simulink model "hcu_main_ADASwEPS"  (Simulink 8.2)
settings: Solver=FixedStepDiscrete  StartTime=0.0  StopTime=inf  FixedStep=0.001  RelTol=1e-3
PostLoadFcn:
  | , if any(exist('dsrtsu_mdlpostloadfcn', 'file') == [2, 3, 6]), try dsrtsu_mdlpostloadfcn('Execute', bdroot); catch fprintf('Error in PostLoadFcn (dsrtsu_mdlpostloadfcn) for model "%s":\n %s\n', bdroot, lasterr); end, end,
values from neighbouring files (symbols this model uses):
  C_TASK_1MS_S = (	C_TICK_TIME_S       )    [hcu_local_hdr.m]    (also in temp_ovrd_values.m = double(	0.001                  ))
  C_TASK_5MS_S = (	C_TICK_TIME_S      	)    [hcu_local_hdr.m]
  ENUM_ADASLFCSTATUS_OFF = uint8(  0  )    [hcu_local_hdr.m]
  ENUM_ADASLFCSTATUS_STANDBY = uint8(  1  )    [hcu_local_hdr.m]
  ENUM_ADASLKASTATUS_ACTIVE = uint8(  2  )    [hcu_local_hdr.m]
  ENUM_ADASLKASTATUS_OFF = uint8(  0  )    [hcu_local_hdr.m]
  ENUM_ADASLKASTATUS_STANDBY = uint8(  1  )    [hcu_local_hdr.m]
  ENUM_EPSMODEREQ_ANGLE = uint8(  1  )    [hcu_local_hdr.m]
  ENUM_EPSMODEREQ_INTERNAL = uint8(  0  )    [hcu_local_hdr.m]
  ENUM_EPSMODEREQ_TORQUE = uint8(  2  )    [hcu_local_hdr.m]
  ENUM_GEARPOSN_1ST = uint8(  1  )    [hcu_local_hdr.m]
  ENUM_GEARPOSN_2ND = uint8(  2  )    [hcu_local_hdr.m]
  ENUM_GEARPOSN_3RD = uint8(  3  )    [hcu_local_hdr.m]
  ENUM_GEARPOSN_4TH = uint8(  4  )    [hcu_local_hdr.m]
  ENUM_GEARPOSN_5TH = uint8(  5  )    [hcu_local_hdr.m]
  ENUM_GEARPOSN_6TH = uint8(  6  )    [hcu_local_hdr.m]
  ENUM_GEARPOSN_PN = uint8(  0  )    [hcu_local_hdr.m]
  ENUM_GEARPOSN_R = uint8(  7  )    [hcu_local_hdr.m]
  FALSE = boolean( 0 )    [hcu_local_hdr.m]
  TRUE = boolean( 1 )    [hcu_local_hdr.m]
undefined symbols (not defined in the file or in its folder): AACC_DistCtrlIMult_X_mps2, AACC_DistCtrlPMult_X_mps2, AACC_GearActual_enum, AACC_SpdCtrlIMult_X_mps2, AACC_SpdCtrlPMult_X_mps2, AACC_VehSpd_kph, AISP_EPSCurrent_pct, AISP_TqASensorDelta_pct, AISP_TqBSensorDelta_pct, ENUM_ACCSTATUS_ACTIVE, ENUM_ACCSTATUS_OFF, ENUM_ACCSTATUS_STANDBY, ENUM_ADASLFCSTATUS_ACTIVE, ENUM_ADASLFCSTATUS_TRANSITION, ENUM_LFCCCONTSTATUS_ACTIVE, ENUM_LFCCCONTSTATUS_NOTAVAIL_TEMP, ENUM_LFCCCONTSTATUS_OFF, ENUM_LFCCCONTSTATUS_READY, ENUM_LFCCCONTSTATUS_TRANSITION, ENUM_LKACCONTSTATUS_ACTIVE, ENUM_LKACCONTSTATUS_NOTAVAIL_TEMP, ENUM_LKACCONTSTATUS_OFF, ENUM_LKACCONTSTATUS_READY, KACC_AcclReqMax_g, KACC_AcclReqMin_g, KACC_ACCSetTimeGapDef1_s, KACC_ACCSetTimeGapDef2_s, KACC_ACCSetTimeGapDef3_s, KACC_ACCSetTimeGapDef4_s, KACC_ACCSetTimeGapDef5_s, KACC_AirDensity_kgpm3, KACC_AirDragCoef_rat, KACC_CommandsOn_flg, KACC_CruzSpdChgTimeThres_s, KACC_DecReqSwOffThres_Nm, KACC_DecReqSwOnThres_Nm, KACC_DistCtrlAdjTime_s, KACC_DistCtrlCalRate_s, KACC_DistCtrlIC_mps2, KACC_DistCtrlIGain_rat, KACC_DistCtrlIMax_mps2, KACC_DistCtrlIMin_mps2, KACC_DistCtrlIRest_flg, KACC_DistCtrlKGain_rat, KACC_DistCtrlPause_flg, KACC_DistCtrlPGain_rat, KACC_FinalDriveEff_pct, KACC_FinalDriveRatio_rat, KACC_FrontalArea_m2, KACC_GearBoxEff_pct, KACC_LongPushSpdChg_kph, KACC_MaxAccSetSpd_kph, KACC_MinAccSetSpd_kph, KACC_SetAllowSpdLim_kph, KACC_SpdCtrlAdjTime_s, KACC_SpdCtrlCalRate_s, KACC_SpdCtrlIC_mps2, KACC_SpdCtrlIGain_rat, KACC_SpdCtrlIMax_mps2, KACC_SpdCtrlIMin_mps2 ... (+26)
libraries: simulink x54, adas_lib x6, rti1401lib_dio_type3 x4, rtimmsu_dsrtlib x3, hcu_lib x2, aeb x1, ddm x1, dfr x1, dgi x1, dhp x1, dinr x1, dip x1
(part 3 of 9)

== system hcu_main_ADASwEPS/Hw_In ==
  trig_Hw_In : TriggerPort  TriggerType=function-call
  ADC_TYPE4_BL1 : rti1401lib_adc_type4/ADC_TYPE4_BL1  DSProperties=struct('RTI',struct('Version',uint32(2),'BlockType',struct('isSLSource',uint8(1),'isSLSink',uint8(1),'isHWSource',uint8(0),'isHWSink',uint8(1),'isSetup',uint8(0),'isInline',uint8(1),'isNonInline',uint8(0),'isInterrupt',uint8(0),'isChannelwise',uint8(1)),'IOBoardType',{{'DS1401','STD','ADCT4'}},'UnitType','ADC','Identifier','ADC','DialogType','ML','BlockSet','NONE','SlaveProcessor','NONE'))  RTIBlockInterface=struct('InputPortsActive',0,'InputPortsWidth',int32(1),'InputPortsDataType',{{'SS_BOOLEAN'}},'InputPortsName',{{'Continue'}},'OutputPortsActive',[1 0],'OutputPortsWidth',int32([1 1]),'OutputPortsDataType',{{'SS_DOUBLE','SS_UINT8'}},'OutputPortsName',{{'ADC','Status'}},'DialogFcn','rti1401stdadct4adcgui','SampleTime',{{-1}},'InitLevel',3,'IconTransparency','on','BlockDisplay',{{['ADC TP4\nModule: 1\nChannel: 1'],'center'}},'BlockName',struct('Token',{{'ADC_TYPE4_BL1'}}))  RTIBlockParameters=struct('ADCSWStartDisable',{{0,'OFF',[0 1]}},'ModuleNo',{{1,'OFF',[1 16]}},'ChannelNo',{{1,'OFF',[1 16]}},'ConversionMode',{{1,'OFF',[1 2]}},'SampleMode',{{1,'OFF',[1 2]}},'TriggerSource',{{1,'OFF',[1 5]}},'EdgePolarity',{{1,'OFF',[1 2]}},'ConversionTriggerSource',{{2,'OFF',[1 6]}},'ConversionEdgePolarity',{{1,'OFF',[1 2]}},'ConversionPeriod',{{1e-06,'OFF',[]}},'ConversionPeriodCheck',{{0,'OFF',[]}},'BurstTriggerSource',{{1,'OFF',[1 6]}},'BurstEdgePolarity',{{1,'OFF',[1 2]}},'BurstSize',{{10,'OFF',[]}},'BurstSizeCheck',{{0,'OFF',[]}},'DataSetOffset',{{0,'OFF',[]}},'DataSetOffsetCheck',{{0,'OFF',[]}},'DataSetLength',{{1,'OFF',[]}},'DataSetLengthCheck',{{0,'OFF',[]}},'ReadMode',{{1,'OFF',[1 2]}},'SampleTime',{{-1,'OFF',[-1 inf]}},'SampleTimeCheck',{{1,'OFF',[]}},'StatusPortEnable',{{0,'OFF',[0 1]}},'VoltageRange',{{1,'OFF',[1 2]}},'TLCFileName',{{'rti1401adc_t4_adc','OFF',[]}})  RTISFcnParameters=struct('ADCSWStartDisable','int32','ModuleNo','int32','ChannelNo','int16','ConversionMode','int16','SampleMode','int16','TriggerSource','int16','EdgePolarity','int16','ConversionTriggerSource','int16','ConversionEdgePolarity','int16','ConversionPeriod','double','BurstTriggerSource','int16','BurstEdgePolarity','int16','BurstSize','int16','DataSetOffset','int16','DataSetLength','int16','ReadMode','int16','SampleTime','double','StatusPortEnable','int16','VoltageRange','int16','TLCFileName','char')  RTIBlockParaDefault=struct('ADCSWStartDisable',0,'ModuleNo',1,'ChannelNo',1,'ConversionMode',1,'SampleMode',1,'TriggerSource',1,'EdgePolarity',1,'ConversionTriggerSource',2,'ConversionEdgePolarity',1,'ConversionPeriod',1e-06,'ConversionPeriodCheck',0,'BurstTriggerSource',1,'BurstEdgePolarity',1,'BurstSize',10,'BurstSizeCheck',0,'DataSetOffset',0,'DataSetOffsetCheck',0,'DataSetLength',1,'DataSetLengthCheck',0,'ReadMode',1,'SampleTime',-1,'SampleTimeCheck',1,'StatusPortEnable',0,'VoltageRange',1,'TLCFileName','rti1401adc_t4_adc')
  Add : Sum
  DIO_TYPE3_ENC_BL1 : rti1401lib_dio_type3/DIO_TYPE3_ENC_BL1  DSProperties=struct('RTI',struct('Version',uint32(2),'BlockType',struct('isSLSource',uint8(1),'isSLSink',uint8(0),'isHWSource',uint8(1),'isHWSink',uint8(0),'isSetup',uint8(0),'isInline',uint8(1),'isNonInline',uint8(0),'isInterrupt',uint8(0),'isChannelwise',uint8(1)),'IOBoardType',{{'DS1401','STD','DIOT3'}},'UnitType','ENC','Identifier','ENC','DialogType','ML','BlockSet','NONE','SlaveProcessor','NONE'))  RTIBlockInterface=struct('OutputPortsWidth',int32([1 1]),'OutputPortsActive',[1 1],'OutputPortsName',{{'Position','Speed'}},'BlockDisplay',{{['DIO TP3 ENCODER\nModule: 1\nPort: 1\nChannel: 9'],'center'}},'IconTransparency','on','InitLevel',3,'DialogFcn','rti1401stddiot3encgui','BlockName',struct('Token',{{'DIO_TYPE3_ENC_BL1'}}))  RTIBlockParameters=struct('ModuleNo',{{1,'OFF',[1 16]}},'PortNo',{{1,'OFF',[1 3]}},'ChannelNo',{{9,'OFF',[1 15]}},'MinPosValue',{{'-2097152','ON',[-2097152 2097151.5]}},'MaxPosValue',{{'2097151.75','ON',[-2097151.75 2097151.75]}},'InitPosValue',{{'0','ON',[-2097152 2097151.75]}},'IndexSetMode',{{1,'OFF',[1 3]}},'IndexPosValue',{{'0','ON',[-2097152 2097151.75]}},'IndexGateMode',{{0,'OFF',[0 1]}},'NoiseFilter',{{1,'OFF',[1 8]}},'BuildCheckIndexMode',{{0,'OFF',[0 1]}},'TLCFileName',{{'rti1401dio_t3_enc','OFF',[]}},'EnableInterrupt',{{0,'OFF',[0 1]}},'TriggerEdgeType',{{1,'OFF',[1 3]}})  RTISFcnParameters=struct('ModuleNo','int32','PortNo','int16','ChannelNo','int16','MinPosValue','double','MaxPosValue','double','InitPosValue','double','IndexSetMode','int16','IndexPosValue','double','IndexGateMode','int16','NoiseFilter','int16','BuildCheckIndexMode','int16','TLCFileName','char','EnableInterrupt','int16','TriggerEdgeType','int32')  RTIBlockParaDefault=struct('ModuleNo',1,'PortNo',1,'ChannelNo',1,'MinPosValue',-2097152,'MaxPosValue',2097151.75,'InitPosValue',0,'IndexSetMode',1,'IndexPosValue',0,'IndexGateMode',0,'NoiseFilter',1,'BuildCheckIndexMode',0,'TLCFileName','rti1401dio_t3_enc','EnableInterrupt',0,'TriggerEdgeType',1)
  DIO_TYPE3_PWM2D_BL1 : rti1401lib_dio_type3/DIO_TYPE3_PWM2D_BL1  DSProperties=struct('RTI',struct('Version',uint32(2),'BlockType',struct('isSLSource',uint8(1),'isSLSink',uint8(0),'isHWSource',uint8(1),'isHWSink',uint8(0),'isSetup',uint8(0),'isInline',uint8(1),'isNonInline',uint8(0),'isInterrupt',uint8(0),'isChannelwise',uint8(1)),'IOBoardType',{{'DS1401','STD','DIOT3'}},'UnitType','PWM','Identifier','PWM2D','DialogType','ML','BlockSet','NONE','SlaveProcessor','NONE'))  RTIBlockInterface=struct('OutputPortsWidth',int32([1 1]),'OutputPortsActive',[1 1],'OutputPortsName',{{'Frequency',['Duty Cycle']}},'BlockDisplay',{{['DIO TP3 PWM2D\nModule: 1\nPort: 1\nChannel: 1'],'center'}},'IconTransparency','on','InitLevel',3,'DialogFcn','rti1401stddiot3pwm2dgui','BlockName',struct('Token',{{'DIO_TYPE3_PWM2D_BL1'}}))  RTIBlockParameters=struct('ModuleNo',{{1,'ON',[1 16]}},'PortNo',{{1,'OFF',[1 3]}},'ChannelNo',{{1,'ON',[1 16]}},'UpdateMode',{{2,'ON',[1 2]}},'FrequencyRange',{{1,'OFF',[1 16]}},'TLCFileName',{{'rti1401dio_t3_pwm2d','OFF',[]}},'EnableInterrupt',{{0,'OFF',[0 1]}},'TriggerEdgeType',{{3,'OFF',[1 3]}})  RTISFcnParameters=struct('ModuleNo','int32','PortNo','int16','ChannelNo','int16','UpdateMode','int16','FrequencyRange','int16','TLCFileName','char','EnableInterrupt','int16','TriggerEdgeType','int32')  RTIBlockParaDefault=struct('ModuleNo',1,'PortNo',1,'ChannelNo',1,'UpdateMode',1,'FrequencyRange',7,'TLCFileName','rti1401dio_t3_pwm2d','EnableInterrupt',0,'TriggerEdgeType',1)
  DIO_TYPE3_PWM2D_BL2 : rti1401lib_dio_type3/DIO_TYPE3_PWM2D_BL1  DSProperties=struct('RTI',struct('Version',uint32(2),'BlockType',struct('isSLSource',uint8(1),'isSLSink',uint8(0),'isHWSource',uint8(1),'isHWSink',uint8(0),'isSetup',uint8(0),'isInline',uint8(1),'isNonInline',uint8(0),'isInterrupt',uint8(0),'isChannelwise',uint8(1)),'IOBoardType',{{'DS1401','STD','DIOT3'}},'UnitType','PWM','Identifier','PWM2D','DialogType','ML','BlockSet','NONE','SlaveProcessor','NONE'))  RTIBlockInterface=struct('OutputPortsWidth',int32([1 1]),'OutputPortsActive',[1 1],'OutputPortsName',{{'Frequency',['Duty Cycle']}},'BlockDisplay',{{['DIO TP3 PWM2D\nModule: 1\nPort: 1\nChannel: 2'],'center'}},'IconTransparency','on','InitLevel',3,'DialogFcn','rti1401stddiot3pwm2dgui','BlockName',struct('Token',{{'DIO_TYPE3_PWM2D_BL1'}}))  RTIBlockParameters=struct('ModuleNo',{{1,'ON',[1 16]}},'PortNo',{{1,'OFF',[1 3]}},'ChannelNo',{{2,'ON',[1 16]}},'UpdateMode',{{2,'ON',[1 2]}},'FrequencyRange',{{1,'OFF',[1 16]}},'TLCFileName',{{'rti1401dio_t3_pwm2d','OFF',[]}},'EnableInterrupt',{{0,'OFF',[0 1]}},'TriggerEdgeType',{{1,'OFF',[1 3]}})  RTISFcnParameters=struct('ModuleNo','int32','PortNo','int16','ChannelNo','int16','UpdateMode','int16','FrequencyRange','int16','TLCFileName','char','EnableInterrupt','int16','TriggerEdgeType','int32')  RTIBlockParaDefault=struct('ModuleNo',1,'PortNo',1,'ChannelNo',1,'UpdateMode',1,'FrequencyRange',7,'TLCFileName','rti1401dio_t3_pwm2d','EnableInterrupt',0,'TriggerEdgeType',1)
  Delay : Delay  DelayLength=1  InitialCondition=1
  Delay1 : Delay  DelayLength=1  InitialCondition=1
  Divide : Product  Inputs=*/
  Divide1 : Product  Inputs=*/
  Divide3 : Product  Inputs=*/
  EPSEncCount_cnt : Constant  Value=36
  EPSGearRatio_rat : Constant  Value=20.5
  Gain1 : Gain  Gain=100
  Gain2 : Gain  Gain=100
  Gain3 : Gain  Gain=100
  Input_Bus : BusCreator  Inputs=6
  Interval Test : simulink/Logic and Bit Operations/Interval Test  IntervalClosedRight=on  uplimit=115  IntervalClosedLeft=on  lowlimit=95  OutDataTypeStr=boolean
  REV2DEG : Gain  Gain=360
  SEC2MIN : Gain  Gain=60
  Switch : Switch  Criteria=u2 ~= 0
  Switch1 : Switch  Criteria=u2 ~= 0
  Terminator3 : Terminator
  Terminator4 : Terminator
  Hw_In : Outport
  wires:
  ADC_TYPE4_BL1/1 -> Gain3/1
  Gain3/1 -> Input_Bus/1  "VHAL_EPSCurrent_pct"
  DIO_TYPE3_PWM2D_BL2/2 -> Gain2/1
  DIO_TYPE3_PWM2D_BL1/2 -> Gain1/1
  Gain1/1 -> Add/1, Switch/1
  DIO_TYPE3_PWM2D_BL1/1 -> Terminator3/1
  DIO_TYPE3_PWM2D_BL2/1 -> Terminator4/1
  Gain2/1 -> Add/2, Switch1/1
  SEC2MIN/1 -> Input_Bus/6  "VHAL_EPSMotorSpd_rpm"
  REV2DEG/1 -> Input_Bus/4, Divide3/1  "VHAL_EPSMotorAng_deg"
  Divide1/1 -> SEC2MIN/1
  Divide/1 -> REV2DEG/1
  EPSEncCount_cnt/1 -> Divide/2, Divide1/2
  DIO_TYPE3_ENC_BL1/2 -> Divide1/1
  DIO_TYPE3_ENC_BL1/1 -> Divide/1
  EPSGearRatio_rat/1 -> Divide3/2
  Divide3/1 -> Input_Bus/5  "VHAL_RelStrAng_deg"
  Input_Bus/1 -> Hw_In/1  "Hw_In"
  Add/1 -> Interval Test/1
  Switch/1 -> Delay/1, Input_Bus/2  "VHAL_TqSensorADuty_pct"
  Switch1/1 -> Delay1/1, Input_Bus/3  "VHAL_TqSensorBDuty_pct"
  Interval Test/1 -> Switch1/2, Switch/2
  Delay/1 -> Switch/3
  Delay1/1 -> Switch1/3

== system hcu_main_ADASwEPS/Hw_Out ==
  OSP_Out : Inport
  trig_Hw_Out : TriggerPort  TriggerType=function-call
  Bus Selector : BusSelector  OutputSignals=DAC_V,EPSDirection_flg
  DAC_TYPE3_M1_C1 : rti1401lib_dac_type3/DAC_TYPE3_M1_C1  ModuleNo=1  ChannelNo=1  VoltageInitValue=0  VoltageTermMode=off  VoltageTermValue=0  Reserved1=[]  Reserved2=[]  Reserved3=[]  Reserved4=[]  DSProperties=struct('RTI',struct('Version',uint32(1),'BlockType',struct('isSLSource',uint8(0),'isSLSink',uint8(1),'isHWSource',uint8(0),'isHWSink',uint8(1),'isSetup',uint8(0),'isInline',uint8(0),'isNonInline',uint8(1),'isInterrupt',uint8(0),'isChannelwise',uint8(1)),'IOBoardType',{{'DS1401','STD','DACT3'}},'UnitType','DAC','Identifier','DAC','DialogType','SL','BlockSet','NONE','SlaveProcessor','NONE'))  RTIBlockInterface=struct('InputPortsActive',1,'BlockDisplay',{{'DAC','center'}},'IconTransparency','off','InitLevel',1,'BlockName',struct('Token',{{'DAC_TYPE3_M','_C'}},'BlockParam',{{'ModuleNo','ChannelNo'}}),'MaskDescription',['Channel-wise write access to the 4 DAC channels'])  RTIBlockParameters=struct('ModuleNo',{{1,'ON',[1 16]}},'ChannelNo',{{1,'ON',[1 4]}},'VoltageInitValue',{{0,'ON',[0 4.5]}},'VoltageTermMode',{{logical(0),'ON',[0 1]}},'VoltageTermValue',{{0,'VoltageTermMode',[0 4.5]}})  RTISFcnParameters=struct('ModuleNo','double','ChannelNo','double','VoltageInitValue','double','VoltageTermMode','double','VoltageTermValue','double')  RTIBlockParaDefault=struct('ModuleNo',1,'ChannelNo',1,'VoltageInitValue',0,'VoltageTermMode',0,'VoltageTermValue',0)
  DIO_TYPE3_BIT_OUT_CH_BL1 : rti1401lib_dio_type3/DIO_TYPE3_BIT_OUT_CH_BL1  DSProperties=struct('RTI',struct('Version',uint32(2),'BlockType',struct('isSLSource',uint8(0),'isSLSink',uint8(1),'isHWSource',uint8(0),'isHWSink',uint8(1),'isSetup',uint8(0),'isInline',uint8(1),'isNonInline',uint8(0),'isInterrupt',uint8(0),'isChannelwise',uint8(1)),'IOBoardType',{{'DS1401','STD','DIOT3'}},'UnitType','BIT','Identifier','BITOUTCH','DialogType','ML','BlockSet','NONE','SlaveProcessor','NONE'))  RTIBlockInterface=struct('InputPortsWidth',int32(1),'InputPortsActive',1,'InputPortsDataType',{{'SS_BOOLEAN'}},'InputPortsName',{{'In'}},'BlockDisplay',{{['DIO TP3 BIT OUT\n Channelwise\nModule: 1\nPort: 1\nChannel: 1'],'center'}},'IconTransparency','on','InitLevel',3,'DialogFcn','rti1401stddiot3bitoutchgui','BlockName',struct('Token',{{'DIO_TYPE3_BIT_OUT_CH_BL1'}}))  RTIBlockParameters=struct('ModuleNo',{{1,'OFF',[1 16]}},'PortNo',{{1,'OFF',[1 3]}},'ChannelNo',{{1,'OFF',[1 16]}},'OutputStateInit',{{0,'OFF',[0 1]}},'TerminationMode',{{0,'OFF',[0 1]}},'OutputStateTermValidate',{{0,'OFF',[0 1]}},'OutputStateTerm',{{0,'OFF',[0 1]}},'SupplyRailsCh',{{[1 1],'OFF',[0 1 0 1]}},'TLCFileName',{{'rti1401dio_t3_bit_out_ch','OFF',[]}},'EnableInterrupt',{{0,'OFF',[0 1]}},'TriggerEdgeType',{{1,'OFF',[1 3]}})  RTISFcnParameters=struct('ModuleNo','int32','PortNo','int16','ChannelNo','int16','SupplyRailsCh','int16','OutputStateInit','int16','TerminationMode','int16','OutputStateTermValidate','int16','OutputStateTerm','int16','TLCFileName','char','EnableInterrupt','int16','TriggerEdgeType','int32')  RTIBlockParaDefault=struct('ModuleNo',1,'PortNo',1,'ChannelNo',1,'OutputStateInit',0,'TerminationMode',0,'OutputStateTermValidate',0,'OutputStateTerm',0,'SupplyRailsCh',[1 1],'TLCFileName','rti1401dio_t3_bit_out_ch','EnableInterrupt',0,'TriggerEdgeType',1)
  Data Type Conversion10 : DataTypeConversion
  Data Type Conversion2 : DataTypeConversion
  wires:
  Data Type Conversion10/1 -> DIO_TYPE3_BIT_OUT_CH_BL1/1
  Data Type Conversion2/1 -> DAC_TYPE3_M1_C1/1
  OSP_Out/1 -> Bus Selector/1
  Bus Selector/1 -> Data Type Conversion2/1  "<DAC_V>"
  Bus Selector/2 -> Data Type Conversion10/1  "<EPSDirection_flg>"

== system hcu_main_ADASwEPS/ISP ==
  Hw_In : Inport
  CAN_In : Inport  Port=2
  trig_ISP : TriggerPort  TriggerType=function-call
  AngleProcessing : Subsystem
  Bus Selector1 : BusSelector  OutputSignals=ABS2.VehSpeed,ADAS1.ADAS_StrAngReq_A,ADAS1.ADAS_StrAngReq,ADAS1.ADAS_LFCTransGain_A,ADAS1.ADAS_LFCTransGain,ABS4.LatAccel,ADAS1.ADAS_StrTqReq_A,ADAS1.ADAS_StrTqReq,ADAS1.ADAS_EPSMode,ADAS1.ADAS_LKAStatus,ADAS1.ADAS_LFCMode,ADAS1.ADAS_LFCStatus
  Bus Selector2 : BusSelector  OutputSignals=VHAL_EPSCurrent_pct
  Bus Selector3 : BusSelector  OutputSignals=VHAL_TqSensorADuty_pct,VHAL_TqSensorBDuty_pct
  Bus Selector4 : BusSelector  OutputSignals=VHAL_RelStrAng_deg
  Bus Selector5 : BusSelector  OutputSignals=VHAL_RelStrAng_deg
  Bus Selector6 : BusSelector  OutputSignals=ABS2.VehSpeed,ABS4.YawRate,ABS4.YawRate_V,ABS3.LR_RawWhlSpeed,ABS3.LR_RawWhlSpeed_V,ABS3.RR_RawWhlSpeed,ABS3.RR_RawWhlSpeed_V
  Bus Selector7 : BusSelector  OutputSignals=VHAL_EPSMotorSpd_rpm,VHAL_RelStrAng_deg
  ISP_Bus : BusCreator  Inputs=21
  KISP_EPSZeroReset_flg : Constant  Value=0
  Logical Operator1 : Logic  Operator=NOT  AllPortsSameDT=off  OutDataTypeStr=boolean
  Logical Operator2 : Logic  Operator=NOT  AllPortsSameDT=off  OutDataTypeStr=boolean
  Logical Operator3 : Logic  Operator=NOT  AllPortsSameDT=off  OutDataTypeStr=boolean
  MISP_EPSCurrent_A : Lookup  InputValues=AISP_EPSCurrent_pct  Table=MISP_EPSCurrent_A  LookUpMeth=Interpolation-Use End Values
      settings: AttributesFormatString="Input=\"%<InputValues>\"\\nOutput=\"%<Table>\""
  PassThrough : Subsystem
  TqProcessing : Subsystem
  ISP_Out : Outport
  wires:
  MISP_EPSCurrent_A/1 -> ISP_Bus/1  "VISP_EPSCurrent_A"
  KISP_EPSZeroReset_flg/1 -> AngleProcessing/1(KISP_EPSZeroReset_flg), TqProcessing/3(KISP_EPSZeroReset_flg)
  Hw_In/1 -> Bus Selector3/1, Bus Selector4/1, [Hw_In], Bus Selector2/1
  ISP_Bus/1 -> ISP_Out/1
  CAN_In/1 -> [CAN_In], Bus Selector1/1
  TqProcessing/1(VISP_EPSTqOnShaft_Nm) -> ISP_Bus/2
  TqProcessing/2(VISP_EPSTqOnShaftValid_flg) -> ISP_Bus/3
  AngleProcessing/1(VISP_StrAng_deg) -> ISP_Bus/4
  AngleProcessing/2(VISP_StrAngValid_flg) -> ISP_Bus/5
  Bus Selector1/1 -> PassThrough/2(VHAL_VehSpd_kph)  "<VehSpeed>"
  Logical Operator2/1 -> AngleProcessing/5(VHAL_YawRateValid_flg)
  Logical Operator3/1 -> AngleProcessing/9(VHAL_RRRawWhlSpdValid_flg)
  Logical Operator1/1 -> AngleProcessing/7(VHAL_LRRawWhlSpdValid_flg)
  PassThrough/1(VISP_StrAngSensorValid_flg) -> ISP_Bus/6
  Bus Selector1/3 -> PassThrough/4(VHAL_StrAngReq_deg)  "<ADAS_StrAngReq>"
  Bus Selector1/2 -> PassThrough/3(VHAL_StrAngReqAppl_flg)  "<ADAS_StrAngReq_A>"
  PassThrough/3(VISP_StrAngReq_deg) -> ISP_Bus/8
  PassThrough/2(VISP_StrAngReqAppl_flg) -> ISP_Bus/7
  PassThrough/4(VISP_VehSpd_kph) -> ISP_Bus/9
  PassThrough/5(VISP_RelStrAng_deg) -> ISP_Bus/10
  Bus Selector1/5 -> PassThrough/6(VHAL_LFCTransGain_rat)  "<ADAS_LFCTransGain>"
  Bus Selector1/4 -> PassThrough/5(VHAL_LFCTransGainAppl_flg)  "<ADAS_LFCTransGain_A>"
  PassThrough/7(VISP_LFCTransGain_rat) -> ISP_Bus/12
  PassThrough/6(VISP_LFCTransGainAppl_flg) -> ISP_Bus/11
  Bus Selector1/6 -> PassThrough/7(VHAL_LatAccel_mps2)  "<LatAccel>"
  PassThrough/8(VISP_LatAccel_mps2) -> ISP_Bus/13
  Bus Selector1/7 -> PassThrough/8(VHAL_StrTqReqAppl_flg)  "<ADAS_StrTqReq_A>"
  Bus Selector1/8 -> PassThrough/9(VHAL_StrTqReq_Nm)  "<ADAS_StrTqReq>"
  PassThrough/9(VISP_StrTqReqAppl_flg) -> ISP_Bus/14
  PassThrough/10(VISP_StrTqReq_Nm) -> ISP_Bus/15
  PassThrough/15(VISP_EPSMotorSpd_rpm) -> ISP_Bus/20
  PassThrough/16(VISP_EPSMotorAng_deg) -> ISP_Bus/21
  Bus Selector2/1 -> MISP_EPSCurrent_A/1  "<VHAL_EPSCurrent_pct>"
  Bus Selector3/1 -> TqProcessing/1(VHAL_TqSensorADuty_pct)  "<VHAL_TqSensorADuty_pct>"
  Bus Selector3/2 -> TqProcessing/2(VHAL_TqSensorBDuty_pct)  "<VHAL_TqSensorBDuty_pct>"
  Bus Selector4/1 -> AngleProcessing/2(VHAL_RelStrAng_deg)  "<VHAL_RelStrAng_deg>"
  Bus Selector5/1 -> PassThrough/1(VHAL_RelStrAng_deg)  "<VHAL_RelStrAng_deg>"
  [Hw_In] -> Bus Selector5/1
  [CAN_In] -> Bus Selector6/1
  Bus Selector6/1 -> AngleProcessing/3(VHAL_VehSpd_kph)  "<VehSpeed>"
  Bus Selector6/2 -> AngleProcessing/4(VHAL_YawRate_degps)  "<YawRate>"
  Bus Selector6/3 -> Logical Operator2/1  "<YawRate_V>"
  Bus Selector6/4 -> AngleProcessing/6(VHAL_LRRawWhlSpd_kph)  "<LR_RawWhlSpeed>"
  Bus Selector6/5 -> Logical Operator1/1  "<LR_RawWhlSpeed_V>"
  Bus Selector6/6 -> AngleProcessing/8(VHAL_RRRawWhlSpd_kph)  "<RR_RawWhlSpeed>"
  Bus Selector6/7 -> Logical Operator3/1  "<RR_RawWhlSpeed_V>"
  [Hw_In] -> Bus Selector7/1
  Bus Selector7/1 -> PassThrough/14(VHAL_EPSMotorSpd_rpm)  "<VHAL_EPSMotorSpd_rpm>"
  Bus Selector7/2 -> PassThrough/15(VHAL_EPSMotorAng_deg)  "<VHAL_RelStrAng_deg>"
  Bus Selector1/9 -> PassThrough/10(VHAL_EPSModeReq_enum)  "<ADAS_EPSMode>"
  Bus Selector1/10 -> PassThrough/11(VHAL_ADASLKAStatus_enum)  "<ADAS_LKAStatus>"
  Bus Selector1/11 -> PassThrough/12(VHAL_ADASLFCMode_enum)  "<ADAS_LFCMode>"
  Bus Selector1/12 -> PassThrough/13(VHAL_ADASLFCStatus_enum)  "<ADAS_LFCStatus>"
  PassThrough/11(VISP_EPSModeReq_enum) -> ISP_Bus/16
  PassThrough/12(VISP_ADASLKAStatus_enum) -> ISP_Bus/17
  PassThrough/13(VISP_ADASLFCMode_enum) -> ISP_Bus/18
  PassThrough/14(VISP_ADASLFCStatus_enum) -> ISP_Bus/19

== system hcu_main_ADASwEPS/OSP ==
  BISP_outputs : Inport
  BEPSS_outputs : Inport  Port=2
  trig_OSP : TriggerPort  TriggerType=function-call
  Abs : Abs
  Bus Creator : BusCreator  Inputs=2
  Bus Selector : BusSelector  OutputSignals=VOSP_MotorDuty_pct
  Compare To Zero : simulink/Logic and Bit Operations/Compare To Zero  relop=>=  OutDataTypeStr=boolean
  Gain3 : Gain  Gain=1/100*4.5
  Negative : Constant  OutDataTypeStr=boolean
  OSP : Subsystem
  Positive : Constant  Value=0  OutDataTypeStr=boolean
  Switch : Switch  Criteria=u2 ~= 0
  OSP_Out : Outport
  BOSP_outputs : Outport  Port=2
  wires:
  Gain3/1 -> Bus Creator/1  "DAC_V"
  Positive/1 -> Switch/1
  Negative/1 -> Switch/3
  Compare To Zero/1 -> Switch/2
  Switch/1 -> Bus Creator/2  "EPSDirection_flg"
  Abs/1 -> Gain3/1
  Bus Creator/1 -> OSP_Out/1  "OSP_Out"
  BEPSS_outputs/1 -> OSP/2(BEPSS_outputs)
  Bus Selector/1 -> Compare To Zero/1, Abs/1  "<VOSP_MotorDuty_pct>"
  OSP/1(BOSP_outputs) -> BOSP_outputs/1, Bus Selector/1
  BISP_outputs/1 -> OSP/1(BISP_outputs)

== system hcu_main_ADASwEPS/RTI Data ==
  RTI Data Store : Subsystem  Tag="struct('private',struct('version',struct('dsVer',uint32(2),'dsVerCreation',uint32(2),'RTI',struct('ver','7.4','type','RTI1401')),'access',struct('type','Model','isPerm',1,'created',['17-Nov-2015 11:37:15'],'modified',['31-Jan-2016 23:13:02'],'location','')),'public',struct('main',struct('data',[]),'sub',struct('name',{{'hcu_main_ADASwEPS'}},'data',{{struct('TH',struct('thTaskInfo',struct('taskType',{'TIMER','HWINT','TMRINT','SWINT','GLINT'},'tasksNumOf',{1,1,0,0,0},'srcIds',{{'TIMERA'},{'BB_BYP_ETHT1M0I0S0'},{},{},{}},'taskNames',{{['Timer Task 1']},{['rti_ethernet_interface_name Interrupt [RX/TX]']},{},{},{}})),'th_tc',struct('dataType',{'TASK','TASK'},'taskGroupId',{'',''},'taskGroupList',{{},{}},'taskSchedulingPolicy',{'FCFS','FCFS'},'taskType',{'TIMER','HWINT'},'blkh',{-1,['hcu_main_ADASwEPS/ETHERNET_UDP_SETUP_BL1/Common Hardware' char(10) 'Interrupt Interface']},'srcId',{'TIMERA','BB_BYP_ETHT1M0I0S0'},'srcSgnName',{['Timer A interrupt'],['BB_BYP_ETH Type 1 Module 1 HW-Int 0 Interrupt 0']},'srcCpuName',{'',''},'taskName',{['Timer Task 1  [0.001] s'],['rti_ethernet_interface_name Interrupt [RX/TX]']},'taskNameDisplayExt',{'',''},'smplTime',{0.001,0},'smplTimeOffs',{0,0},'hasFixedPriority',{0,0},'priority',{1,2},'hasFixedOvc',{0,0},'ovcType',{1,1},'ovcMax',{1,1}),'tc_th',struct('dataType',{'TASK','TASK'},'taskGroupId',{'',''},'taskGroupList',{{},{}},'taskSchedulingPolicy',{'FCFS','FCFS'},'taskType',{'TIMER','HWINT'},'blkh',{-1,['hcu_main_ADASwEPS/ETHERNET_UDP_SETUP_BL1/Common Hardware' char(10) 'Interrupt Interface']},'srcId',{'TIMERA','BB_BYP_ETHT1M0I0S0'},'srcSgnName',{['Timer A interrupt'],['BB_BYP_ETH Type 1 Module 1 HW-Int 0 Interrupt 0']},'srcCpuName',{'',''},'taskName',{['Timer Task 1  [0.001] s'],['rti_ethernet_interface_name Interrupt [RX/TX]']},'taskNameDisplayExt',{'',''},'smplTime',{0.001,0},'smplTimeOffs',{0,0},'hasFixedPriority',{0,0},'priority',{1,2},'hasFixedOvc',{0,0},'ovcType',{1,1},'ovcMax',{1,1}))}})))"  mask(RTI_DATA_STORE){}
      mask help:
      | RTI Data Store Block. This block is used by RTI to store internal model dependent data. Deleting this block will result in data loss.
      |
      | NEVER DELETE, COPY, OR MODIFY THIS BLOCK!
      mask Help:
      | RTI Data Store Block. This block is used by RTI to store internal model dependent data. Deleting this block will result in data loss.
      | 
      | NEVER DELETE, COPY, OR MODIFY THIS BLOCK!
      mask Display: text(0.5, 0.5, ' ', 'HorizontalAlignment', 'center');

== system hcu_main_ADASwEPS/RTICANMM ControllerSetup ==
  VariationInput : Inport
  Reset : Inport  Port=2
  ModelClose : Subsystem  mask(RTICANMMModelClose){}
  RTICANMMCHANNEL_TLC : S-Function  FunctionName=rticanmm_tlc_adv  Parameters=1401,1,1,0,500,14011143421  EnableBusSupport=off  mask(RTICANMMCHANNEL_TLC){}
  Variation_DTC : DataTypeConversion  SaturateOnIntegerOverflow=on  RndMeth=Zero
  sfcn : S-Function  InitFcn=rticanmm_initfcn(gcb, 'SFCNs')  FunctionName=RTICANMM_SETUP_CAN_1  EnableBusSupport=off
      mask init:
      | rticanmm_initfcn(gcb, 'SFCNs')
  wires:
  Reset/1 -> sfcn/2
  VariationInput/1 -> Variation_DTC/1
  Variation_DTC/1 -> sfcn/1

== system hcu_main_ADASwEPS/RTICANMM ControllerSetup1 ==
  VariationInput : Inport
  Reset : Inport  Port=2
  ModelClose : Subsystem  mask(RTICANMMModelClose){}
  RTICANMMCHANNEL_TLC : S-Function  FunctionName=rticanmm_tlc_adv  Parameters=1401,1,2,0,500,14011243421  EnableBusSupport=off  mask(RTICANMMCHANNEL_TLC){}
  Variation_DTC : DataTypeConversion  SaturateOnIntegerOverflow=on  RndMeth=Zero
  sfcn : S-Function  InitFcn=rticanmm_initfcn(gcb, 'SFCNs')  FunctionName=RTICANMM_SETUP_CAN_2  EnableBusSupport=off
      mask init:
      | rticanmm_initfcn(gcb, 'SFCNs')
  wires:
  Reset/1 -> sfcn/2
  VariationInput/1 -> Variation_DTC/1
  Variation_DTC/1 -> sfcn/1

== system hcu_main_ADASwEPS/RTICANMM GeneralSetup ==
  ModelClose : Subsystem  mask(RTICANMMModelClose){}
  TRC Exclusion : rtimmsu_dsrtlib/TRC Exclusion

== system hcu_main_ADASwEPS/User2CAN1__ ==
  BOSP_outputs : Inport
  BOUTP_outputs : Inport  Port=2  OutDataTypeStr=Bus: BOUTP_outputs
  ADAS1 : Subsystem
  ADAS2 : Subsystem
  ADAS3 : Subsystem
  ADAS4 : Subsystem
  ADAS5 : Subsystem
  EPAS2 : Subsystem
  EPAS3 : Subsystem
  SAS1 : Subsystem
  buscreator : BusCreator  Inputs=8
  out : Outport
  wires:
  ADAS1/1(out) -> buscreator/1  "ADAS1"
  ADAS2/1(out) -> buscreator/2  "ADAS2"
  ADAS3/1(out) -> buscreator/3  "ADAS3"
  ADAS4/1(out) -> buscreator/4  "ADAS4"
  ADAS5/1(out) -> buscreator/5  "ADAS5"
  EPAS2/1(out) -> buscreator/6  "EPAS2"
  EPAS3/1(out) -> buscreator/7  "EPAS3"
  SAS1/1(out) -> buscreator/8  "SAS1"
  buscreator/1 -> out/1  "CAN"
  BOUTP_outputs/1 -> ADAS1/1(BOUTP_outputs), ADAS2/1(BOUTP_outputs), ADAS3/1(BOUTP_outputs), ADAS5/1(BOUTP_outputs), ADAS4/1(BOUTP_outputs)
  BOSP_outputs/1 -> SAS1/1(BOSP_outputs), EPAS3/1(BOSP_outputs), EPAS2/1(BOSP_outputs)

== system hcu_main_ADASwEPS/User2RTICANMM MainBlock_ ==
  CAN1_Rx : Inport
  ABS2_C : Subsystem
  ABS4_C : Subsystem
  SAS1_C : Subsystem
  SpeedInformation : Subsystem
  YawRateInformation : Subsystem
  buscreator : BusCreator  Inputs=5
  out : Outport
  wires:
  ABS2_C/1(out) -> buscreator/1  "ABS2_C"
  ABS4_C/1(out) -> buscreator/2  "ABS4_C"
  SAS1_C/1(out) -> buscreator/3  "SAS1_C"
  SpeedInformation/1(out) -> buscreator/4  "SpeedInformation"
  YawRateInformation/1(out) -> buscreator/5  "YawRateInformation"
  buscreator/1 -> out/1  "CAN"
  CAN1_Rx/1 -> YawRateInformation/1(CAN1_Rx), SpeedInformation/1(CAN1_Rx), SAS1_C/1(CAN1_Rx), ABS4_C/1(CAN1_Rx), ABS2_C/1(CAN1_Rx1)

== system hcu_main_ADASwEPS/APPH/ACC ==
  BDINR_outputs : Inport  OutDataTypeStr=Bus: BDINR_outputs
  BMCT_outputs : Inport  Port=2  OutDataTypeStr=Bus: BMCT_outputs
  BAEB_outputs : Inport  Port=3  OutDataTypeStr=Bus: BAEB_outputs
  trig_ACC : TriggerPort  TriggerType=function-call
  ACC : Subsystem
  Bus Creator : BusCreator  Inputs=8  OutDataTypeStr=Bus: BACC_outputs
  Bus Selector1 : BusSelector  OutputSignals=VDINR_DriverBrakPedalOn_flg,VDINR_VehSpd_kph,VDINR_ACCOnVCU_flg,VDINR_ACCResSpdIncVCU_flg,VDINR_ACCSetSpdDecVCU_flg,VDINR_ACCTimeGapIncVCU_flg,VDINR_ACCTimeGapDecVCU_flg,VDINR_NowGearPosn_enum,VDINR_EngSpd_erpm,VDINR_DefMaxACCSetSpeed_kph
  Bus Selector2 : BusSelector  OutputSignals=VAEB_AEBActive_flg
  Bus Selector3 : BusSelector  OutputSignals=VMCT_MCTPositionX_m,VMCT_MCTRelVelocityX_mps,VMCT_MCTInPath_flg
  model_info : Subsystem  LoadFcn=slcm LoadBlock;  InitFcn=slcm('UpdateAllCMBlocksInThisModelInit')  mask(CMBlock){InitialSaveTempField=, InitialBlockCM=None, BlockCM=None, Frame=on, SaveTempField=, DisplayStringWithTags=$Id: aeb.mdl 800 2014-08-28 03:32:11Z JuneXmas $, MaskDisplayString=$Id: aeb.mdl 800 2014-08-28 03:32:11Z JuneXmas $, HorizontalTextAlignment=Center, LeftAlignmentValue=0.5, SourceBlockDiagram=hcu_main_ADASwEPS, TagMaxNumber=20, CMTag1=, CMTag2=, CMTag3=, CMTag4=, CMTag5=, CMTag6=, CMTag7=, CMTag8=, CMTag9=, CMTag10=, CMTag11=, CMTag12=, CMTag13=, CMTag14=, CMTag15=, CMTag16=, CMTag17=, CMTag18=, CMTag19=, CMTag20=}
      mask help: This block allows revision control information to be displayed within the model.
      settings: CopyFcn=slcm CopyBlock;  DeleteFcn=slcm Cancel;  PostSaveFcn=slcm('UpdateAllCMBlocksInThisModel')  NameChangeFcn=slcm Rename;  OpenFcn=slcm
      mask Display: text(str2num(LeftAlignmentValue), 0.5, MaskDisplayString, 'HorizontalAlignment', HorizontalTextAlignment)
  BACC_outputs : Outport  OutDataTypeStr=Bus: BACC_outputs
  wires:
  BDINR_outputs/1 -> Bus Selector1/1
  Bus Creator/1 -> BACC_outputs/1  "BACC_outputs"
  Bus Selector1/1 -> ACC/1(VDINR_DriverBrakPedalOn_flg)  "<VDINR_DriverBrakPedalOn_flg>"
  Bus Selector1/2 -> ACC/2(VDINR_VehSpd_kph)  "<VDINR_VehSpd_kph>"
  Bus Selector1/3 -> ACC/3(VDINR_ACCOnVCU_flg)  "<VDINR_ACCOnVCU_flg>"
  Bus Selector1/4 -> ACC/4(VDINR_ACCResSpdIncVCU_flg)  "<VDINR_ACCResSpdIncVCU_flg>"
  Bus Selector1/5 -> ACC/5(VDINR_ACCSetSpdDecVCU_flg)  "<VDINR_ACCSetSpdDecVCU_flg>"
  Bus Selector1/6 -> ACC/6(VDINR_ACCTimeGapIncVCU_flg)  "<VDINR_ACCTimeGapIncVCU_flg>"
  Bus Selector1/7 -> ACC/7(VDINR_ACCTimeGapDecVCU_flg)  "<VDINR_ACCTimeGapDecVCU_flg>"
  ACC/1(VACC_ACCStatus_enum) -> Bus Creator/1
  Bus Selector1/8 -> ACC/8(VDINR_NowGearPosn_enum)  "<VDINR_NowGearPosn_enum>"
  Bus Selector1/9 -> ACC/9(VDINR_EngSpd_rpm)  "<VDINR_EngSpd_erpm>"
  ACC/7(VACC_DecReq_mps2) -> Bus Creator/7
  ACC/6(VACC_TqReqAppl_flg) -> Bus Creator/6
  ACC/8(VACC_DecReqAppl_flg) -> Bus Creator/8
  ACC/5(VACC_TqReq_Nm) -> Bus Creator/5
  BMCT_outputs/1 -> Bus Selector3/1
  Bus Selector1/10 -> ACC/10(VDINR_DefMaxACCSetSpeed_kph)  "<VDINR_DefMaxACCSetSpeed_kph>"
  ACC/2(VACC_ACCSetTimeGap_enum) -> Bus Creator/2
  ACC/3(VACC_ACCSetTimeGapTmp_enum) -> Bus Creator/3
  ACC/4(VACC_ACCSetSpd_kph) -> Bus Creator/4
  Bus Selector3/2 -> ACC/12(VMCT_MCTRelVelocityX_mps)  "<VMCT_MCTRelVelocityX_mps>"
  Bus Selector3/1 -> ACC/11(VMCT_MCTPositionX_m)  "<VMCT_MCTPositionX_m>"
  Bus Selector3/3 -> ACC/13(VMCT_MCTInPath_flg)  "<VMCT_MCTInPath_flg>"
  BAEB_outputs/1 -> Bus Selector2/1
  Bus Selector2/1 -> ACC/14(VAEB_AEBActive_flg)  "<VAEB_AEBActive_flg>"

== system hcu_main_ADASwEPS/CAN1/ModelClose ==
